simulink model "EPS_sim_test_v6b"  (R2023b)
settings: Solver=FixedStepAuto  StartTime=0.0  StopTime=tsimulation  FixedStep=delta_t  MaxStep=10  RelTol=1e-3
values from neighbouring files (symbols this model uses):
  ADCS =     [RWinfo.mat]
undefined symbols (not defined in the file or in its folder): Bat, EN, EPS, FIPEX, GPS, OBC, OCS, PL, UHF
libraries: simulink x4
settings Model: Creator=Ricardo  LastModifiedBy=lricc
settings SolverCC: AlgebraicLoopSolver=TrustRegion
settings OptimizationCC: ReuseModelBlockBuffer=off
settings DebuggingCC: UnconnectedInputMsg=warning  UnconnectedOutputMsg=warning  UnconnectedLineMsg=warning
settings ModelReferenceCC: EnableRefExpFcnMdlSchedulingChecks=on
settings SFSimCC: CustomCodeUndefinedFunction=UseInterfaceOnly
settings RTWCC: DLArmComputeVersion=19.05

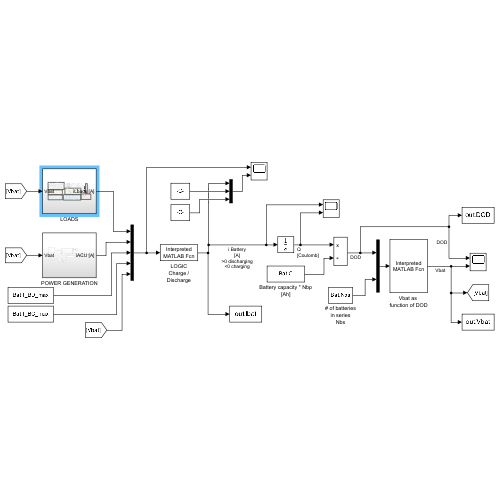
[thumbnail: Simulink's stored preview of the top-level diagram]
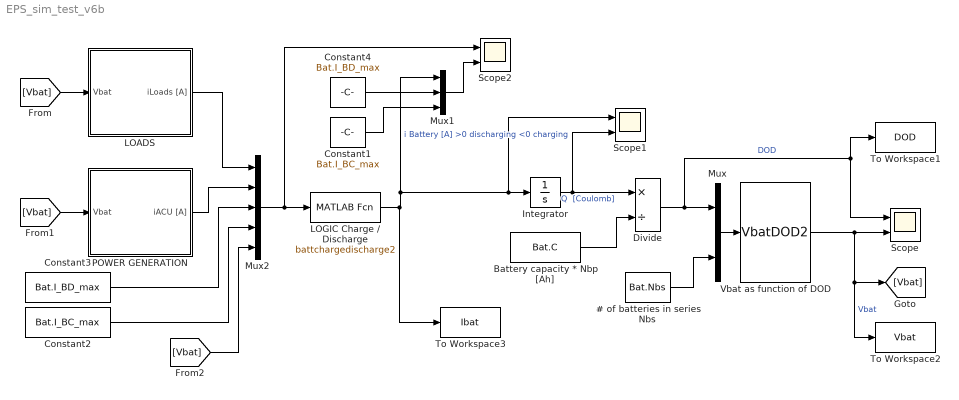
== system EPS_sim_test_v6b ==
  # of batteries in series Nbs : Constant  Value=Bat.Nbs
  Battery capacity * Nbp [Ah] : Constant  Value=Bat.C
  Constant1 : Constant  Value=Bat.I_BC_max
  Constant2 : Constant  Value=Bat.I_BC_max
  Constant3 : Constant  Value=Bat.I_BD_max
  Constant4 : Constant  Value=Bat.I_BD_max
  Divide : Product  Inputs=*/
  Integrator : Integrator  InitialCondition=Bat.DOD_0*Bat.C
  LOADS : Subsystem
  LOGIC Charge / Discharge : MATLABFcn  MATLABFcn=battchargedischarge2
  Mux : Mux  Inputs=2
  Mux1 : Mux  Inputs=3
  Mux2 : Mux  Inputs=5
  POWER GENERATION : Subsystem
  Scope : Scope  NumInputPorts=2
  Scope1 : Scope  NumInputPorts=2
  Scope2 : Scope  NumInputPorts=2
  To Workspace1 : ToWorkspace  VariableName=DOD  SaveFormat=Timeseries  SampleTime=-1
  To Workspace2 : ToWorkspace  VariableName=Vbat  SaveFormat=Timeseries  SampleTime=-1
  To Workspace3 : ToWorkspace  VariableName=Ibat  SaveFormat=Timeseries  SampleTime=-1
  Vbat as function of DOD : MATLABFcn  MATLABFcn=VbatDOD2
  wires:
  Mux/1 -> Vbat as function of DOD/1
  # of batteries in series Nbs/1 -> Mux/2
  Vbat as function of DOD/1 -> [Vbat], To Workspace2/1, Scope/2  "Vbat"
  Divide/1 -> To Workspace1/1, Scope/1, Mux/1  "DOD"
  Integrator/1 -> Scope1/2, Divide/1  "Q  [Coulomb]"
  Battery capacity * Nbp [Ah]/1 -> Divide/2
  [Vbat] -> LOADS/1(Vbat)
  POWER GENERATION/1(iACU [A]) -> Mux2/2
  [Vbat] -> POWER GENERATION/1(Vbat)
  LOADS/1(iLoads [A]) -> Mux2/1
  Mux2/1 -> LOGIC Charge / Discharge/1, Scope2/1
  Constant3/1 -> Mux2/3
  Constant2/1 -> Mux2/4
  LOGIC Charge / Discharge/1 -> To Workspace3/1, Mux1/1, Scope1/1, Integrator/1  "i Battery [A] >0 discharging <0 charging"
  [Vbat] -> Mux2/5
  Mux1/1 -> Scope2/2
  Constant4/1 -> Mux1/2
  Constant1/1 -> Mux1/3

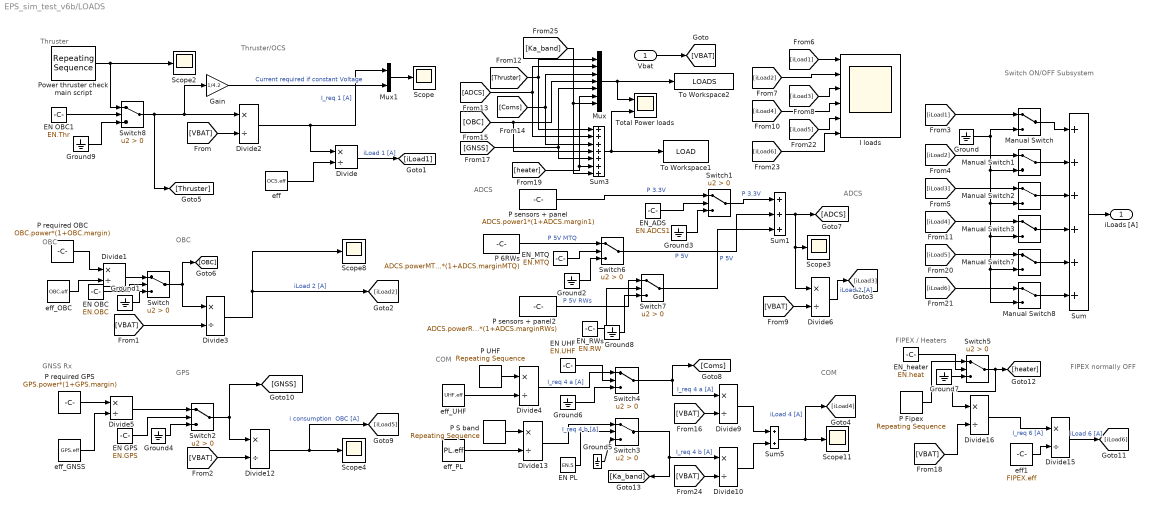
== system EPS_sim_test_v6b/LOADS ==
  note: Switch
      | ON/OFF
      | Subsystem
  note: FIPEX / Heaters
  note: COM
  note: ADCS
  note: OBC
  note: Thruster
  note: Thruster/OCS
  note: OBC
  note: ADCS
  note: COM
  note: GPS
  note: GNSS Rx
  note: FIPEX
      | normally
      | OFF
  Vbat : Inport
  Divide{,1..6,9..10,12..13,15..16} (13 alike) : Product  Inputs=*/
  EN GPS : Constant  Value=EN.GPS
  EN OBC : Constant  Value=EN.OBC
  EN OBC1 : Constant  Value=EN.Thr
  EN PL : Constant  Value=EN.S
  EN UHF : Constant  Value=EN.UHF
  EN_ADS : Constant  Value=EN.ADCS1
  EN_MTQ : Constant  Value=EN.MTQ
  EN_RWs : Constant  Value=EN.RW
  EN_heater : Constant  Value=EN.heat
  Gain : Gain  Gain=1/4.2
  Ground{,1..9} (10 alike) : Ground
  I loads : Scope  NumInputPorts=6
  Manual Switch{,1..3,7..8} (6 alike) : ManualSwitch
  Mux : Mux  Inputs=7
  Mux1 : Mux  Inputs=2
  P 6RWs : Constant  Value=ADCS.powerMTQ/ADCS.effMTQ *(1+ADCS.marginMTQ)
  P Fipex : simulink/Sources/Repeating Sequence  rep_seq_t=FIPEX.t_Fi  rep_seq_y=FIPEX.p_Fi*(1+FIPEX.margin)
  "P S band " : simulink/Sources/Repeating Sequence  rep_seq_t=PL.t_tx_S  rep_seq_y=PL.p_tx_S*(1+PL.margin)
  "P UHF " : simulink/Sources/Repeating Sequence  rep_seq_t=UHF.t_tx_UHF  rep_seq_y=UHF.p_tx_UHF*(1+UHF.margin)
  P required GPS : Constant  Value=GPS.power*(1+GPS.margin)
  P required OBC : Constant  Value=OBC.power*(1+OBC.margin)
  P sensors + panel : Constant  Value=ADCS.power1*(1+ADCS.margin1)
  P sensors + panel2 : Constant  Value=ADCS.powerRWs/ADCS.effRW *(1+ADCS.marginRWs)
  Power thruster check main script : simulink/Sources/Repeating Sequence  rep_seq_t=OCS.t_thr  rep_seq_y=OCS.p_thr*(1+OCS.margin)
  Scope{,2..4,8,11} (6 alike) : Scope
  Sum : Sum  Inputs=++++++
  Sum1 : Sum  Inputs=+++
  Sum3 : Sum  Inputs=+++++++
  Sum5 : Sum
  Switch{,1..8} (9 alike) : Switch  Criteria=u2 > Threshold  SaturateOnIntegerOverflow=off  InputSameDT=off
  To Workspace1 : ToWorkspace  VariableName=LOAD  SaveFormat=Timeseries  SampleTime=-1
  To Workspace2 : ToWorkspace  VariableName=LOADS  SaveFormat=Timeseries  SampleTime=-1
  Total Power loads : Scope  NumInputPorts=2
  eff : Constant  Value=OCS.eff
  eff1 : Constant  Value=FIPEX.eff
  eff_GNSS : Constant  Value=GPS.eff
  eff_OBC : Constant  Value=OBC.eff
  eff_PL : Constant  Value=PL.eff
  eff_UHF : Constant  Value=UHF.eff
  iLoads [A] : Outport
  wires:
  Gain/1 -> Mux1/2  "Current required if constant Voltage"
  Divide2/1 -> Divide/1, Mux1/1  "I_req 1 [A]"
  [VBAT] -> Divide3/2
  Vbat/1 -> [VBAT]
  [VBAT] -> Divide2/2
  Sum/1 -> iLoads [A]/1
  Mux1/1 -> Scope/1
  eff_OBC/1 -> Divide1/2
  Switch8/1 -> [Thruster], Gain/1, Divide2/1
  eff/1 -> Divide/2
  Divide/1 -> [iLoad1]  "iLoad 1 [A]"
  Manual Switch/1 -> Sum/1
  Manual Switch1/1 -> Sum/2
  Manual Switch2/1 -> Sum/3
  [iLoad2] -> I loads/2
  [iLoad1] -> I loads/1
  [iLoad3] -> I loads/3
  [iLoad4] -> I loads/4
  Manual Switch3/1 -> Sum/4
  "P UHF "/1 -> Divide4/1
  [iLoad4] -> Manual Switch3/1
  [iLoad3] -> Manual Switch2/1
  [iLoad2] -> Manual Switch1/1
  [iLoad1] -> Manual Switch/1
  Ground/1 -> Manual Switch/2, Manual Switch8/2, Manual Switch7/2, Manual Switch3/2, Manual Switch2/2, Manual Switch1/2
  Mux/1 -> To Workspace2/1, Total Power loads/1
  [Thruster] -> Sum3/1, Mux/1
  [ADCS] -> Sum3/2, Mux/2
  [Coms] -> Sum3/3, Mux/3
  [OBC] -> Sum3/4, Mux/4
  [heater] -> Mux/6, Sum3/6
  Sum3/1 -> Total Power loads/2, To Workspace1/1
  Divide12/1 -> [iLoad5], Scope4/1  "i consumption  OBC [A]"
  [VBAT] -> Divide12/2
  eff_GNSS/1 -> Divide5/2
  [GNSS] -> Sum3/5, Mux/5
  eff1/1 -> Divide15/2
  Divide15/1 -> [iLoad6]  "iLoad 6 [A]"
  P Fipex/1 -> Switch5/1
  Divide16/1 -> Divide15/1  "I_req 6 [A]"
  [VBAT] -> Divide16/2
  Switch5/1 -> Divide16/1, [heater]
  Manual Switch7/1 -> Sum/5
  Manual Switch8/1 -> Sum/6
  [iLoad6] -> Manual Switch8/1
  [iLoad5] -> Manual Switch7/1
  [iLoad5] -> I loads/5
  [iLoad6] -> I loads/6
  Switch1/1 -> Sum1/1  "P 3.3V"
  P required OBC/1 -> Divide1/1
  Switch/1 -> Divide3/1, [OBC]
  Divide3/1 -> Scope8/1, [iLoad2]  "iLoad 2 [A]"
  P required GPS/1 -> Divide5/1
  Switch2/1 -> [GNSS], Divide12/1
  "P S band "/1 -> Divide13/1
  eff_PL/1 -> Divide13/2
  Switch4/1 -> [Coms], Divide9/1  "I_req 4 a [A]"
  Switch3/1 -> Divide10/1, [Ka_band]  "I_req 4 b [A]"
  eff_UHF/1 -> Divide4/2
  [VBAT] -> Divide9/2
  [VBAT] -> Divide10/2
  Divide10/1 -> Sum5/2
  Divide9/1 -> Sum5/1
  [VBAT] -> Divide6/2
  Divide6/1 -> [iLoad3]  "iLoad 2 [A]"
  Divide1/1 -> Switch/1
  EN OBC/1 -> Switch/2
  Ground1/1 -> Switch/3
  Ground4/1 -> Switch2/3
  EN GPS/1 -> Switch2/2
  Divide5/1 -> Switch2/1
  Ground5/1 -> Switch3/3
  EN PL/1 -> Switch3/2
  EN UHF/1 -> Switch4/2
  Ground6/1 -> Switch4/3
  Divide4/1 -> Switch4/1  "I_req 4 a [A]"
  Divide13/1 -> Switch3/1  "I_req 4 b [A]"
  Ground7/1 -> Switch5/3
  EN_heater/1 -> Switch5/2
  Ground3/1 -> Switch1/3
  EN_ADS/1 -> Switch1/2
  P sensors + panel/1 -> Switch1/1  "P 3.3V"
  Ground9/1 -> Switch8/3
  EN OBC1/1 -> Switch8/2
  Power thruster check main script/1 -> Scope2/1, Switch8/1
  Sum5/1 -> [iLoad4], Scope11/1  "iLoad 4 [A]"
  [Ka_band] -> Sum3/7, Mux/7
  P 6RWs/1 -> Switch6/1  "P 5V MTQ"
  EN_MTQ/1 -> Switch6/2
  Ground2/1 -> Switch6/3
  Ground8/1 -> Switch7/3
  EN_RWs/1 -> Switch7/2
  P sensors + panel2/1 -> Switch7/1  "P 5V RWs"
  Sum1/1 -> Divide6/1, Scope3/1, [ADCS]
  Switch6/1 -> Sum1/2  "P 5V"
  Switch7/1 -> Sum1/3  "P 5V"

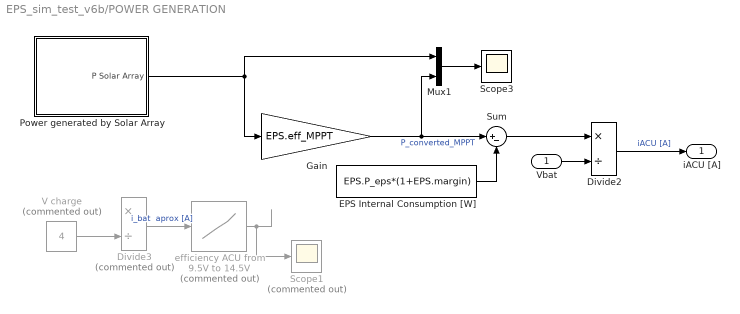
== system EPS_sim_test_v6b/POWER GENERATION ==
  Vbat : Inport
  Divide2 : Product  Inputs=*/
  Divide3 : Product  Commented=on  Inputs=*/
  EPS Internal Consumption [W] : Constant  Value=EPS.P_eps*(1+EPS.margin)
  Gain : Gain  Gain=EPS.eff_MPPT
  Mux1 : Mux  Inputs=2
  Power generated by Solar Array : Subsystem
  Scope1 : Scope  Commented=on
  Scope3 : Scope
  Sum : Sum  Inputs=|+-
  V charge : Constant  Commented=on  Value=4
  efficiency ACU from 9.5V to 14.5V : Lookup_n-D  Commented=on  NumberOfTableDimensions=1  BreakpointsForDimension1=[0,0.13,0.16,0.236,0.4187,0.654,0.684,0.745,0.801,0.9372,1.046,1.16,1.21,1.5,1.66,2,4]  Table=[0.905,0.928,0.9296,0.9296,0.9337,0.9296,0.9296,0.9296,0.9275,0.9275,0.9254,0.9254,0.9234,0.9193,0.9193,0.9134,0.9134]  InternalRulePriority=Speed  RndMeth=Simplest
  iACU [A] : Outport
  wires:
  Divide2/1 -> iACU [A]/1  "iACU [A]"
  Mux1/1 -> Scope3/1
  Vbat/1 -> Divide2/2
  efficiency ACU from 9.5V to 14.5V/1 -> Scope1/1
  Gain/1 -> Sum/1, Mux1/2  "P_converted_MPPT"
  Sum/1 -> Divide2/1
  EPS Internal Consumption [W]/1 -> Sum/2
  Divide3/1 -> efficiency ACU from 9.5V to 14.5V/1  "i_bat  aprox [A]"
  V charge/1 -> Divide3/2
  Power generated by Solar Array/1(P Solar Array) -> Gain/1, Mux1/1

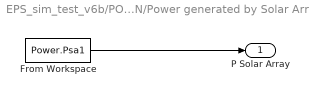
== system EPS_sim_test_v6b/POWER GENERATION/Power generated by Solar Array ==
  From Workspace : FromWorkspace  VariableName=Power.Psa1
  P Solar Array : Outport
  wires:
  From Workspace/1 -> P Solar Array/1
